simulink model "Copy_of_NewApproach"  (R2022a)
settings: Solver=VariableStepAuto  StartTime=0.0  StopTime=43  FixedStep=0.01  RelTol=1e-3
undefined symbols (not defined in the file or in its folder): B, Spline, X, Y, Z
libraries: sm_lib x171, nesl_utility x58, fl_lib x31, sh_lib x13, robotcorelib x6, slpidlib x4
(part 1 of 6)
settings Model: Creator=Jakob  LastModifiedBy=Jakob

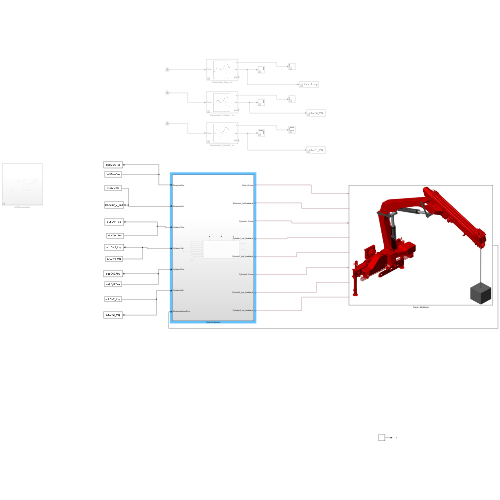
[thumbnail: Simulink's stored preview of the top-level diagram]
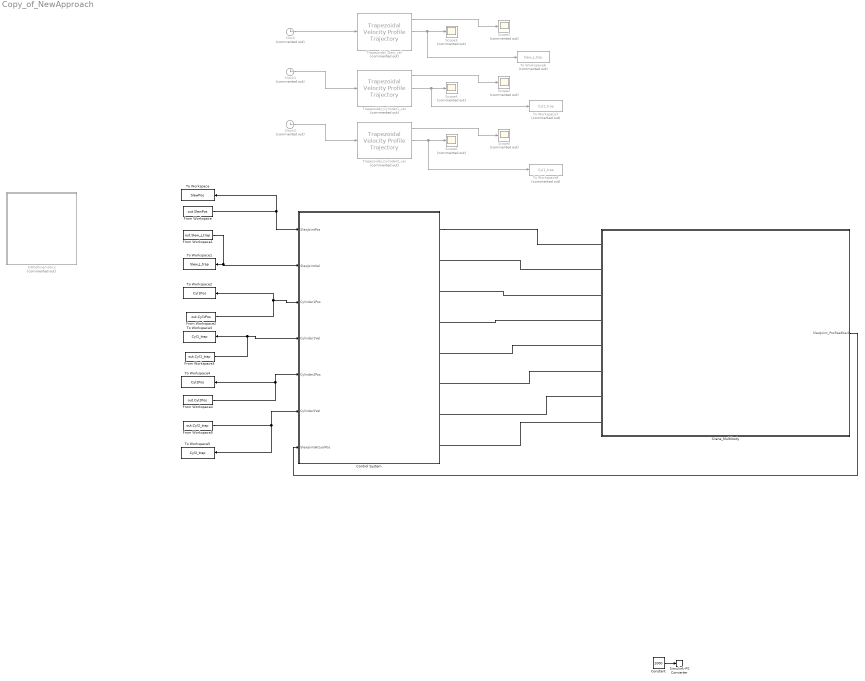
== system Copy_of_NewApproach ==
  Clock : Clock  Commented=on
  Clock1 : Clock  Commented=on
  Clock2 : Clock  Commented=on
  Constant : Constant  Value=1000
  Control System : Subsystem
  Crane_Multibody : Subsystem
      mask Display: image('$imagefile'); % Use "Edit Image" on toolstrip to change.
  From Workspace : FromWorkspace  VariableName=out.SlewPos
  From Workspace1 : FromWorkspace  VariableName=out.Slew_J_trap
  From Workspace2 : FromWorkspace  VariableName=out.Cyl1Pos
  From Workspace3 : FromWorkspace  VariableName=out.Cyl1_trap
  From Workspace4 : FromWorkspace  VariableName=out.Cyl2Pos
  From Workspace5 : FromWorkspace  VariableName=out.Cyl2_trap
  HOG/Kinematics : Subsystem  Commented=on
  Scope{1..6} (6 alike) : Scope  Commented=on
  Simulink-PS Converter : nesl_utility/Simulink-PS Converter  PhysicalDomain=network_engine_domain  SubClassName=ps_input  LeftPortType=input  RightPortType=output  PseudoPeriodic=off  Frequencies=[]  NoiseDistribution=none  NoiseParameters=[]  Unit=1  AffineConversion=off  FilteringAndDerivatives=provide  SimscapeFilterOrder=1  InputFilterTimeConstant=0.001  UdotUserProvided=0
      settings: SourceProductBaseCode=SS,PW,VE
  To Workspace : ToWorkspace  VariableName=SlewPos  SaveFormat=Timeseries  SampleTime=-1
      settings: Decimation=10
  To Workspace1 : ToWorkspace  VariableName=Slew_J_trap  SaveFormat=Timeseries  SampleTime=-1
  To Workspace2 : ToWorkspace  VariableName=Cyl1Pos  SaveFormat=Timeseries  SampleTime=-1
  To Workspace3 : ToWorkspace  VariableName=Cyl1_trap  SaveFormat=Timeseries  SampleTime=-1
  To Workspace4 : ToWorkspace  VariableName=Cyl2Pos  SaveFormat=Timeseries  SampleTime=-1
  To Workspace5 : ToWorkspace  VariableName=Cyl2_trap  SaveFormat=Timeseries  SampleTime=-1
  To Workspace6 : ToWorkspace  Commented=on  VariableName=Slew_J_trap  SaveFormat=Timeseries  SampleTime=-1
      settings: Decimation=10
  To Workspace7 : ToWorkspace  Commented=on  VariableName=Cyl2_trap  SaveFormat=Timeseries  SampleTime=-1
      settings: Decimation=10
  To Workspace8 : ToWorkspace  Commented=on  VariableName=Cyl1_trap  SaveFormat=Timeseries  SampleTime=-1
      settings: Decimation=10
  Trapezoidal_Cylinder1_vel : robotcorelib/Trapezoidal Velocity Profile Trajectory  Commented=on  WaypointSource=Internal  Waypoints=[0.540702, 0.423835, 0.709263, 0.578643]  NumParams=1  Parameter1=End Time  Parameter2=Peak Velocity  ParameterSource=Internal  PeakVelocity=[ 0.016,0.075, 0.005 ]  Acceleration=[ 1; 2 ]  EndTime=[14.33]  AccelTime=[ 1; 2 ]  SimulateUsing=Interpreted execution
      settings: SourceProductBaseCode=RO,NV,RR,UV
  Trapezoidal_Cylinder2_vel : robotcorelib/Trapezoidal Velocity Profile Trajectory  Commented=on  WaypointSource=Internal  Waypoints=[0.499310, 0.6532636, 0.6930204, 0.679982]  NumParams=1  Parameter1=End Time  Parameter2=Peak Velocity  ParameterSource=Internal  PeakVelocity=[ 0.016,0.075, 0.005 ]  Acceleration=[ 1; 2 ]  EndTime=[14.33]  AccelTime=[ 1; 2 ]  SimulateUsing=Interpreted execution
      settings: SourceProductBaseCode=RO,NV,RR,UV
  Trapezoidal_Slew_vel : robotcorelib/Trapezoidal Velocity Profile Trajectory  Commented=on  WaypointSource=Internal  Waypoints=[-0.2682, -0.16, -0.0622, -0.0245]  NumParams=1  Parameter1=End Time  Parameter2=Peak Velocity  ParameterSource=Internal  PeakVelocity=[ 0.016,0.075, 0.005 ]  Acceleration=[ 1; 2 ]  EndTime=[14.33]  AccelTime=[ 1; 2 ]  SimulateUsing=Interpreted execution
      settings: SourceProductBaseCode=RO,NV,RR,UV
  wires:
  Constant/1 -> Simulink-PS Converter/1
  From Workspace5/1 -> To Workspace5/1, Control System/6(Cylinder2Vel)
  From Workspace4/1 -> Control System/5(Cylinder2Pos), To Workspace4/1
  From Workspace3/1 -> Control System/4(Cylinder1Vel), To Workspace3/1
  From Workspace2/1 -> To Workspace2/1, Control System/3(Cylinder1Pos)
  From Workspace1/1 -> Control System/2(SlewJointVel), To Workspace1/1
  From Workspace/1 -> Control System/1(SlewJointPos), To Workspace/1
  Crane_Multibody/1(SlewJoint_PosFeedback) -> Control System/7(SlewJointActualPos)
  Clock/1 -> Trapezoidal_Slew_vel/1
  Trapezoidal_Slew_vel/2 -> To Workspace6/1, Scope3/1
  Trapezoidal_Slew_vel/1 -> Scope1/1
  Clock1/1 -> Trapezoidal_Cylinder1_vel/1
  Trapezoidal_Cylinder1_vel/1 -> Scope2/1
  Trapezoidal_Cylinder1_vel/2 -> To Workspace7/1, Scope4/1
  Clock2/1 -> Trapezoidal_Cylinder2_vel/1
  Trapezoidal_Cylinder2_vel/1 -> Scope5/1
  Trapezoidal_Cylinder2_vel/2 -> To Workspace8/1, Scope6/1
  connections:
  Control System/RConn1 -- Crane_Multibody/LConn1
  Crane_Multibody/LConn2 -- Control System/RConn2
  Crane_Multibody/LConn3 -- Control System/RConn3
  Crane_Multibody/LConn4 -- Control System/RConn4
  Crane_Multibody/LConn5 -- Control System/RConn5
  Crane_Multibody/LConn6 -- Control System/RConn6
  Crane_Multibody/LConn7 -- Control System/RConn7
  Crane_Multibody/LConn8 -- Control System/RConn8

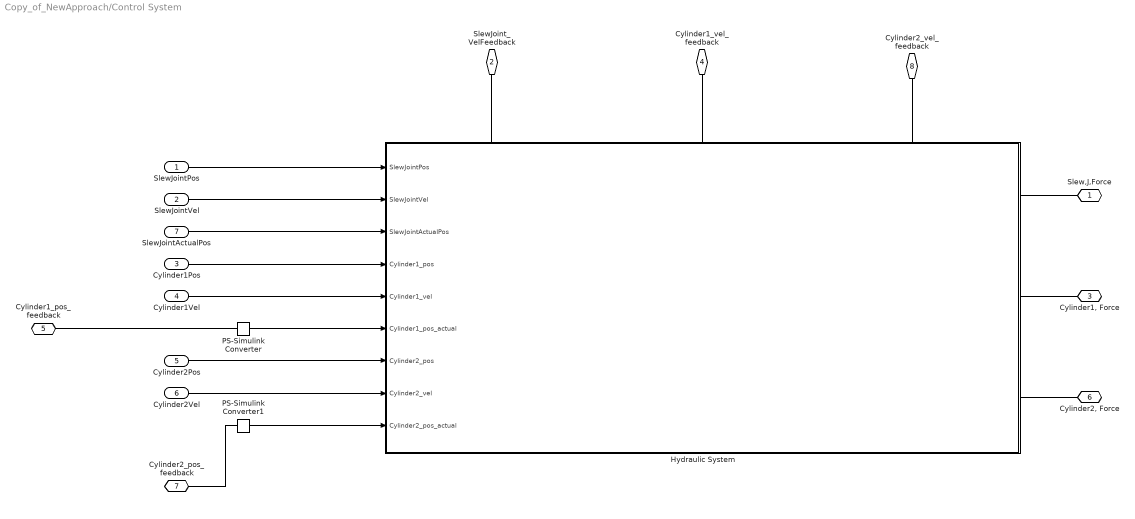
== system Copy_of_NewApproach/Control System ==
  SlewJointPos : Inport
  SlewJointVel : Inport  Port=2
  Cylinder1Pos : Inport  Port=3
  Cylinder1Vel : Inport  Port=4
  Cylinder2Pos : Inport  Port=5
  Cylinder2Vel : Inport  Port=6
  SlewJointActualPos : Inport  Port=7
  Hydraulic System : Subsystem
      settings: PortSchema="{\"entries\":[{\"content\":{\"sides\":[{\"content\":{\"connectorIds\":[\"In1\",\"In2\",\"In3\",\"In4\",\"In5\",\"In6\",\"In7\",\"In8\",\"In9\"]},\"type\":\"ConnectorPlacement.EquallySpacedRectSide\",\"uuid\":\"c66543fa-198c-4f99-bad8-b3fba23087d9\"},{\"content\":{\"connectorIds\":[\"RConn1\",\"RConn2\",\"RConn3\"],\"side\":\"RIGHT\"},\"type\":\"ConnectorPlacement.EquallySpacedRectSide\",\"uuid\":\"68dc06a0-8d9d-4ec7-aacb-b23d2e6fbaba\"},{\"content\":{\"connectorIds\":[\"LConn1\",\"LConn2\",\"LConn3\"],\"side\":\"TOP\"},\"type\":\"ConnectorPlacement.EquallySpacedRectSide\",\"uuid\":\"7cecdc53-4657-4882-ad34-35515944277c\"}]},\"type\":\"ConnectorPlacement.EquallySpacedConnector\",\"uuid\":\"472e1db7-f81a-4c73-97d6-ba992d4f136f\"}],\"packageUris\":[\"http://schema.mathworks.com/mf0/Connector/R2020b\"],\"version\":\"1.0\"}"
  PS-Simulink Converter : nesl_utility/PS-Simulink Converter  PhysicalDomain=network_engine_domain  SubClassName=ps_output  LeftPortType=input  RightPortType=output  PseudoPeriodic=off  Frequencies=[]  VectorFormat=inherit  Unit=inherit  AffineConversion=off
      settings: SourceProductBaseCode=SS,PW,VE
  PS-Simulink Converter1 : nesl_utility/PS-Simulink Converter  PhysicalDomain=network_engine_domain  SubClassName=ps_output  LeftPortType=input  RightPortType=output  PseudoPeriodic=off  Frequencies=[]  VectorFormat=inherit  Unit=inherit  AffineConversion=off
      settings: SourceProductBaseCode=SS,PW,VE
  Slew,J,Force : PMIOPort  Side=Right
  SlewJoint_VelFeedback : PMIOPort  Port=2  Side=Right
  "Cylinder1, Force" : PMIOPort  Port=3  Side=Right
  Cylinder1_vel_feedback : PMIOPort  Port=4  Side=Right
  Cylinder1_pos_feedback : PMIOPort  Port=5  Side=Right
  "Cylinder2, Force" : PMIOPort  Port=6  Side=Right
  Cylinder2_pos_feedback : PMIOPort  Port=7  Side=Right
  Cylinder2_vel_feedback : PMIOPort  Port=8  Side=Right
  wires:
  SlewJointPos/1 -> Hydraulic System/1(SlewJointPos)
  SlewJointVel/1 -> Hydraulic System/2(SlewJointVel)
  SlewJointActualPos/1 -> Hydraulic System/3(SlewJointActualPos)
  Cylinder1Pos/1 -> Hydraulic System/4(Cylinder1_pos)
  Cylinder1Vel/1 -> Hydraulic System/5(Cylinder1_vel)
  Cylinder2Pos/1 -> Hydraulic System/7(Cylinder2_pos)
  Cylinder2Vel/1 -> Hydraulic System/8(Cylinder2_vel)
  PS-Simulink Converter/1 -> Hydraulic System/6(Cylinder1_pos_actual)
  PS-Simulink Converter1/1 -> Hydraulic System/9(Cylinder2_pos_actual)
  connections:
  Slew,J,Force/RConn1 -- Hydraulic System/RConn1
  SlewJoint_VelFeedback/RConn1 -- Hydraulic System/LConn1
  Cylinder1_vel_feedback/RConn1 -- Hydraulic System/LConn2
  "Cylinder1, Force"/RConn1 -- Hydraulic System/RConn2
  Cylinder2_vel_feedback/RConn1 -- Hydraulic System/LConn3
  "Cylinder2, Force"/RConn1 -- Hydraulic System/RConn3
  Cylinder1_pos_feedback/RConn1 -- PS-Simulink Converter/LConn1
  PS-Simulink Converter1/LConn1 -- Cylinder2_pos_feedback/RConn1
